simulink model "Uncertain_System"  (R2024b)
settings: Solver=ode45  StartTime=0.0  StopTime=60  RelTol=1e-6  AbsTol=1e-8
settings Model: Creator=LAPTOPASADI  LastModifiedBy=LAPTOPASADI

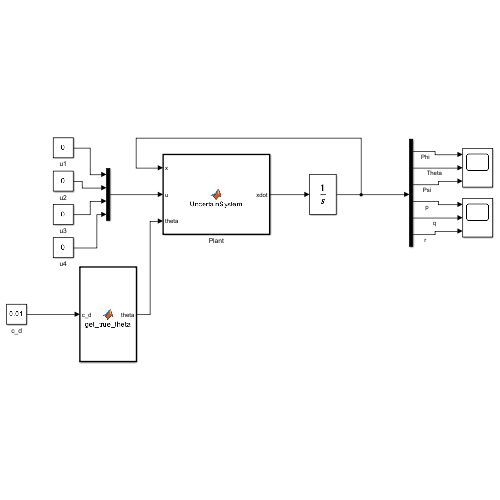
[thumbnail: Simulink's stored preview of the top-level diagram]
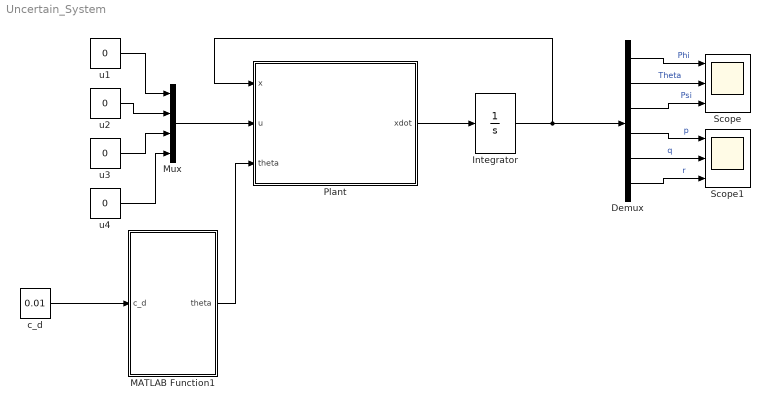
== system Uncertain_System ==
  Demux : Demux  Outputs=6
  Integrator : Integrator  InitialCondition=[0.0873;0.0524;0.1745;0.5;-0.3;0.2]
  MATLAB Function1 : MATLAB Function  TreatAsAtomicUnit=on
  Mux : Mux
  Plant : MATLAB Function  TreatAsAtomicUnit=on
  Scope : Scope  NumInputPorts=3
  Scope1 : Scope  NumInputPorts=3
  c_d : Constant  Value=0.01
  u{1..4} (4 alike) : Constant  Value=0
  wires:
  Plant/1(xdot) -> Integrator/1
  c_d/1 -> MATLAB Function1/1(c_d)
  u1/1 -> Mux/1
  Mux/1 -> Plant/2(u)
  u2/1 -> Mux/2
  MATLAB Function1/1(theta) -> Plant/3(theta)
  u3/1 -> Mux/3
  u4/1 -> Mux/4
  Demux/6 -> Scope1/3  "r"
  Demux/1 -> Scope/1  "Phi"
  Demux/5 -> Scope1/2  "q"
  Demux/4 -> Scope1/1  "p"
  Integrator/1 -> Demux/1, Plant/1(x)
  Demux/3 -> Scope/3  "Psi"
  Demux/2 -> Scope/2  "Theta"

== matlab function Uncertain_System/Plant ==
  data: x input; u input; xdot output; theta input
function xdot = UncertainSystem(x, u, theta)
%#codegen
% MATLAB Function block for  Uncertain_System.slx.
% Inputs : x (6), u (4), theta (6)
% Output : xdot (6) so that  xdot = f0(x) + F(x)*theta + g(x)*u.

    Ixx = 0.0043;  Iyy = 0.0142;  Izz = 0.0176;  Ixz = 1e-4;
    dcg = 0.175;   hcg = 0.085;   d_over_b = 1.2e-6 / 3.13e-5;

    I = [ Ixx, 0, -Ixz;  0, Iyy, 0;  -Ixz, 0, Izz];
    B_alloc = [0, 0,   dcg,        d_over_b;
               0, hcg, 0,          0;
               0, 0,   d_over_b,  -dcg];

    phi = x(1);  th = x(2);
    p   = x(4);  q  = x(5);  r = x(6);
    omega = [p; q; r];

    cphi = cos(phi);  sphi = sin(phi);
    cth  = cos(th);   sth  = sin(th);
    if abs(cth) < 1e-6, cth = sign(cth + 1e-6)*1e-6; end
    tth = sth/cth;

    J = [1, sphi*tth, cphi*tth;
         0, cphi,    -sphi;
         0, sphi/cth, cphi/cth];

    F_omega = [ p*q, -q*r, 0,    0,           0,   -p;
                0,    0,   p*r, -(p^2 - r^2), 0,   -q;
               -q*r,  0,   0,    0,           p*q, -r];

    f0    = [J*omega; 0; 0; 0];
    F_reg = [zeros(3,6); F_omega];
    g     = [zeros(3,4); I \ B_alloc];

    xdot = f0 + F_reg*theta + g*u;
end

== matlab function Uncertain_System/MATLAB Function1 ==
  data: c_d input; theta output
function theta = get_true_theta(c_d)
    
    Ixx = 0.0043;
    Iyy = 0.0142;
    Izz = 0.0176;
    Ixz = 0.0001;

    Gam = Ixx * Izz - Ixz^2;

    Gam1 = (Ixz * (Ixx - Iyy + Izz)) / Gam;
    Gam2 = (Izz * (Izz - Iyy) + Ixz^2) / Gam;
    Gam5 = (Izz - Ixx) / Iyy;
    Gam6 = Ixz / Iyy;
    Gam7 = ((Ixx - Iyy) * Ixx + Ixz^2) / Gam;

    theta = [Gam1; Gam2; Gam5; Gam6; Gam7; c_d];

end
